simulink model "lpfilter"  (Simulink 7.3)
settings: Solver=ode45  StartTime=0.0  StopTime=100.0  RelTol=1e-3
settings Model: Creator=MAHESH  LastModifiedBy=Achyut

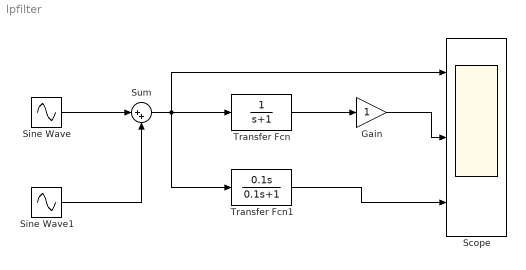
== system lpfilter ==
  Gain : Gain  ParameterDataType=fixdt(1, 16)  ParameterScaling=2^0  OutDataType=fixdt(1, 16)  OutScaling=2^0
  Scope : Scope  NumInputPorts=3
      settings: YMin=-5~-5~-5  YMax=5~5~5
  Sine Wave : Sin  Amplitude=5  Bias=0  Frequency=1  Phase=0  Samples=10  SampleTime=0  Offset=0
  Sine Wave1 : Sin  Amplitude=1  Bias=0  Frequency=10  Phase=0  Samples=10  SampleTime=0  Offset=0
  Sum : Sum  Inputs=|++  OutDataType=fixdt(1, 16)  OutScaling=2^0
  Transfer Fcn : TransferFcn  Denominator=[1 1]
  Transfer Fcn1 : TransferFcn  Numerator=[0.1 0]  Denominator=[0.1 1]
  wires:
  Sine Wave/1 -> Sum/1
  Sum/1 -> Transfer Fcn/1, Scope/1, Transfer Fcn1/1
  Transfer Fcn/1 -> Gain/1
  Sine Wave1/1 -> Sum/2
  Gain/1 -> Scope/2
  Transfer Fcn1/1 -> Scope/3
